simulink model "d_003_uc"  (Simulink 5.1)
settings: Solver=ode45  StartTime=0.0  StopTime=10.0  RelTol=1e-3
libraries: fm_lib x4
settings Model: Creator=fmilano  LastModifiedBy=fmilano  ExtModeAutoUpdateStatusClock=off  SignalLoggingName=logsout  BooleanDataType=on  RTWOptions="-aEnforceIntegerDowncast=1 -aFoldNonRolledExpr=1 -aInlineInvariantSignals=1 -aInlineParameters=0 -aLocalBlockOutputs=1 -aRollThreshold=5 -aZeroInternalMemoryAtStartup=1 -aZeroExternalMemoryAtStartup=1 -aInitFltsAndDblsToZero=1 -aForceBlockIOInitOptimize=0 -aGenerateReport=0 -aGenCodeOnly=0 -aRTWVerbose=1 -aIncludeHyperlinkInReport=0 -aLaunchReport=0 -aGenerateTraceInfo=0  -aForceParamTrailComments=0 -aGenerateComments=1 -aIgnoreCustomStorageClasses=1 -aIncHierarchyInIds=0 -aMaxRTWIdLen=31 -aShowEliminatedStatements=0 -aIncDataTypeInIds=0 -aInsertBlockDesc=0 -aIgnoreTestpoints=0 -aSimulinkBlockComments=1 -aInlinedPrmAccess=\"Literals\"  -aSuppressErrorStatus=0 -aModelReferenceCompliant=1 -aParenthesesLevel=\"Nominal\" -aModelStepFunctionPrototypeControlCompliant=0 -aPortableWordSizes=0 -aParMdlRefBuildCompliant=1 -aSupportNonInlinedSFcns=1 -aSupportContinuousTime=1 -aSupportComplex=1 -aSupportNonFinite=1 -aSupportAbsoluteTime=1 -aMultiwordLength=2048 -aTargetPreCompLibLocation=\"\" -aTargetLibSuffix=\"\" -aTargetFunctionLibrary=\"ANSI_C\" -aTargetFcnLib=\"ansi_tfl_tmw.mat\" -aMultiInstanceERTCode=0 -aLogVarNameModifier=\"rt_\" -aERTFirstTimeCompliant=0 -aIsPILTarget=0 -aCombineOutputUpdateFcns=0 -aGenerateASAP2=0 -aGenerateClassInterface=0 -aGenerateTestInterfaces=0 -aGenerateSampleERTMain=0 -aGenerateFullHeader=1 -aUtilityFuncGeneration=\"Auto\" -aIncludeFileDelimiter=\"Auto\" -aIncludeMdlTerminateFcn=1 -aPurelyIntegerCode=0 -aAutosarCompliant=0 -aERTCustomFileBanners=0 -aRTWCAPIStates=0 -aRTWCAPIParams=0 -aRTWCAPISignals=0 -aMatFileLogging=1 -aCompOptLevelCompliant=0 -aCPPClassGenCompliant=0 -aExtModeIntrfLevel=\"Level1\" -aExtModeMexFile=\"ext_comm\" -aExtModeTransport=0 -aExtModeStaticAllocSize=1000000 -aExtModeTesting=0 -aExtModeStaticAlloc=0 -aExtMode=0 -aERTMultiwordLength=256 -aERTMultiwordTypeDef=\"System defined\"  -aGenerateTraceInfo=0 -aIgnoreTestpoints=0 -aGenerateTraceInfo=0 -aGenerateTraceInfo=0 -aGenerateTraceInfo=0 -aGenerateTraceInfo=0 -aPrefixModelToSubsysFcnNames=1"

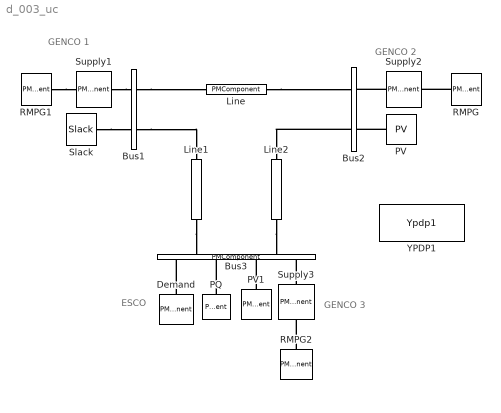
== system d_003_uc ==
  note: GENCO 1
  note: GENCO 2
  note: GENCO 3
  note: ESCO
  Bus1 : PMComponent  Tag=PSATblock  Description=Connection  PhysicalDomain=psatdomain  LeftPortType=p1  RightPortType=p1  LConnTagsString=__newl0|__newl1  RConnTagsString=__newr0|__newr1  mask(Bus){in=2, out=2, p2q=400, p3_4q=[1.00   0.00], p5q=1, p6q=1}
      mask prompts: in "Number of inputs:"; out "Number of outputs:"; p2q "Voltage Rating [kV]"; p3_4q "Voltage initial guess [p.u.  rad]"; p5q "Area number"; p6q "Region number"
      mask help: Bus block.
      mask init:
      | fm_inout
      mask CallbackString: ||||fm_block|
      mask Display: plot([0 1 1 0 0],[0 0 1 1 0])
  Bus2 : PMComponent  Tag=PSATblock  Description=Connection  PhysicalDomain=psatdomain  LeftPortType=p1  RightPortType=p1  LConnTagsString=__newl0|__newl1  RConnTagsString=__newr0|__newr1  mask(Bus){in=2, out=2, p2q=400, p3_4q=[1.00   0.00], p5q=2, p6q=1}
      mask prompts: in "Number of inputs:"; out "Number of outputs:"; p2q "Voltage Rating [kV]"; p3_4q "Voltage initial guess [p.u.  rad]"; p5q "Area number"; p6q "Region number"
      mask help: Bus block.
      mask init:
      | fm_inout
      mask CallbackString: ||||fm_block|
      mask Display: plot([0 1 1 0 0],[0 0 1 1 0])
  Bus3 : PMComponent  Tag=PSATblock  Description=Connection  Orientation=down  PhysicalDomain=psatdomain  LeftPortType=p1  RightPortType=p1  LConnTagsString=__newl0|__newl1  RConnTagsString=__newr0|__newr1|__newr2|__newr3  mask(Bus){in=2, out=4, p2q=400, p3_4q=[1.00  0.00], p5q=3, p6q=1}
      mask prompts: in "Number of inputs:"; out "Number of outputs:"; p2q "Voltage Rating [kV]"; p3_4q "Voltage initial guess [p.u.  rad]"; p5q "Area number"; p6q "Region number"
      mask help: Bus block.
      mask init:
      | fm_inout
      mask CallbackString: ||||fm_block|
      mask Display: plot([0 1 1 0 0],[0 0 1 1 0])
  Demand : PMComponent  Tag=PSATblock  Description=OPF & CPF  Orientation=down  PhysicalDomain=psatdomain  LeftPortType=p1  RightPortType=p1  LConnTagsString=__newl0  mask(Demand){p2q=100, p3q=1.00, p4q=0.60, p5_6q=[1.00  1.00], p8_9_10q=[0.00  0  0.00], p11_12_13q=[0.00  0.00  0.00], p14q=off, p15q=0, p16_17q=[0 0], out=0, p18q=on}
      mask prompts: p2q "Power Rating [MVA]"; p3q "Active Power [p.u.]"; p4q "Reactive Power [p.u.]"; p5_6q "Max and Min Power Demand [p.u.  p.u.]"; p8_9_10q "Cost = a + b*P + c*P^2 [$/h, $/MWh, $/(MW)^2 h]"; p11_12_13q "Cost = a + b*Q + c*Q^2 [$/h, $/MVArh, $/(MVAr)^2 h]"; p14q "Allow Unit Commitment"; p15q "Tie Breaking Cost [$/h]"; p16_17q "Up and down congestion costs [$/h $/h]"; out "Number of Output Signals"; p18q "Connected"
      mask help: This block defines a constant power load for bifurcation and market studies.
      mask init:
      | fm_inout;
      | [xs,ys]=fm_draw('$');
      mask StyleString: edit,edit,edit,edit,edit,edit,checkbox,edit,edit,popup(0|1),checkbox
      mask CallbackString: ||||||||||fm_block
      mask Display:
      | plot([ 1.0000    -0.5   -0.5  1],[ 0    0.866    -0.866    0])
      | color('blue')
      | plot(0.6*xs,0.6*ys)
  Line : PMComponent  Tag=PSATblock  Description=Power Flow  PhysicalDomain=psatdomain  LeftPortType=p1  RightPortType=p1  LConnTagsString=__newl0  RConnTagsString=__newr0  mask(Line){p3_4_5q=[100  400  60], p6q=0, p8q=0, p9q=0.10, p10q=0, p13_14_15q=[0.4  0.4  0.0], p16q=on}
      mask prompts: p3_4_5q "Power, Voltage and Frequency Ratings [MVA, kV, Hz]"; p6q "Length of line [km] (0 for p.u. parameters)"; p8q "Resistance [p.u. (Ohms/km)]"; p9q "Reactance [p.u. (H/km)]"; p10q "Susceptance [p.u. (F/km)]"; p13_14_15q "Imax, Pmax and Smax [p.u., p.u., p.u.]"; p16q "Connected"
      mask help: This block defines a pi model for a tree phase line.
      mask init:
      | [xp,yp] = fm_draw('pi');
      mask CallbackString: ||||||fm_block
      mask Display:
      | plot([-1  1  1 -1 -1],[-0.2 -0.2 0.2 0.2 -0.2])
      | color('blue')
      | plot(0.35*xp,0.2*yp)
  Line1 : PMComponent  Tag=PSATblock  Description=Power Flow  Orientation=down  PhysicalDomain=psatdomain  LeftPortType=p1  RightPortType=p1  LConnTagsString=__newl0  RConnTagsString=__newr0  mask(Line){p3_4_5q=[100  400  60], p6q=0, p8q=0, p9q=0.10, p10q=0, p13_14_15q=[0.4  0.4  0.0], p16q=on}
      mask prompts: p3_4_5q "Power, Voltage and Frequency Ratings [MVA, kV, Hz]"; p6q "Length of line [km] (0 for p.u. parameters)"; p8q "Resistance [p.u. (Ohms/km)]"; p9q "Reactance [p.u. (H/km)]"; p10q "Susceptance [p.u. (F/km)]"; p13_14_15q "Imax, Pmax and Smax [p.u., p.u., p.u.]"; p16q "Connected"
      mask help: This block defines a pi model for a tree phase line.
      mask init:
      | [xp,yp] = fm_draw('pi');
      mask CallbackString: ||||||fm_block
      mask Display:
      | plot([-1  1  1 -1 -1],[-0.2 -0.2 0.2 0.2 -0.2])
      | color('blue')
      | plot(0.35*xp,0.2*yp)
  Line2 : fm_lib/Power Flow/Line  Tag=PSATblock  Description=Power Flow  Orientation=down  PhysicalDomain=psatdomain  SubClassName=unknown  LeftPortType=p1  RightPortType=p1  LConnTagsString=__newl0  RConnTagsString=__newr0  p3_4_5q="[100  400  60]"  p6q=0  p8q=0  p9q=0.10  p10q=0  p13_14_15q="[0.4  0.4  0.0]"  p16q=on
  PQ : PMComponent  Tag=PSATblock  Description=Power Flow  Orientation=down  PhysicalDomain=psatdomain  LeftPortType=p1  RightPortType=p1  LConnTagsString=__newl0  mask(PQ){p2_3q=[100  400], p4_5q=[1.0 0.6], p6_7q=[1.2  0.8], p8q=on, p9q=on}
      mask prompts: p2_3q "Power and Voltage Ratings [MVA, kV]"; p4_5q "Active and Reactive Powers [p.u.  p.u.]"; p6_7q "Maximum and Minimum Allowable Voltage [p.u.   p.u.]"; p8q "Allow conversion to impendance for min & max voltage"; p9q "Connected"
      mask help:
      | This block defines a constant power load:
      |
      | P = Pcost.
      | Q = Qcost.
      mask CallbackString: |||fm_block|fm_block
      mask Display: plot([1 -0.5 -0.5 1],[0 0.866 -0.866 0])
  PV : fm_lib/Power Flow/PV  Tag=PSATblock  Description=Power Flow  Orientation=left  PhysicalDomain=psatdomain  SubClassName=unknown  LeftPortType=p1  RightPortType=p1  RConnTagsString=__newr0  p2_3q="[100  400]"  p4q=0.4  p5q=1.00  p6_7q="[0.8  -0.2]"  p8_9q="[1.1  0.9]"  p10q=1  p11q=on
  PV1 : PMComponent  Tag=PSATblock  Description=Power Flow  Orientation=up  PhysicalDomain=psatdomain  LeftPortType=p1  RightPortType=p1  RConnTagsString=__newr0  mask(PV){p2_3q=[100  400], p4q=0.4, p5q=1.00, p6_7q=[0.8  -0.2], p8_9q=[1.1  0.9], p10q=1, p11q=on}
      mask prompts: p2_3q "Power and Voltage Ratings [MVA, kV]"; p4q "Active Power [p.u.]"; p5q "Voltage Magnitude [p.u.]"; p6_7q "Qmax & Qmin [p.u.  p.u.]"; p8_9q "Vmax & Vmin [p.u.  p.u.]"; p10q "Loss Participation Factor"; p11q "Connected"
      mask help:
      | This block defines a PV bus for load flow studies:
      |
      | P = Pcost.
      | V = Vdes.
      mask init:
      | [x,y] = fm_draw('circle');
      | [xp,yp] = fm_draw('P');
      mask CallbackString: ||||||fm_block
      mask Display:
      | plot(x,y)
      | color('blue')
      | plot(0.3*xp-0.35,0.6*yp,[0.1 0.3 0.5],[0.3 -0.3 0.3])
  RMPG : PMComponent  Tag=PSATblock  Description=OPF & CPF  Orientation=left  PhysicalDomain=psatdomain  LeftPortType=p1  RightPortType=p1  RConnTagsString=__newr0  mask(Rmpg){p2q=100, p3_4q=[0.1  0.1], p5_6q=[2 2], p7_8q=[5 0], p9q=1, p10q=on}
      mask prompts: p2q "Power Rating [MVA]"; p3_4q "Ramp Up and Down Rates [p.u./h  p.u./h]"; p5_6q "Minimum Up and Down Times [h  h]"; p7_8q "Numbers of period up and down at initial time [h  h]"; p9q "Start Up Cost [$]"; p10q "Conneted"
      mask help: This block defines ramping parameters for generators for market studies.
      mask init:
      | [x,y] = fm_draw('circle');
      mask CallbackString: |||||fm_block
      mask Display:
      | plot(x,y)
      | color('blue')
      | plot([-0.5 0.5],[-0.4 -0.4],[-0.4 -0.4],[-0.45 0.4],[-0.4 0],[-0.5 0.3],[0 0.4],[0.3 0.3])
  RMPG1 : PMComponent  Tag=PSATblock  Description=OPF & CPF  PhysicalDomain=psatdomain  LeftPortType=p1  RightPortType=p1  RConnTagsString=__newr0  mask(Rmpg){p2q=100, p3_4q=[0.05 0.05], p5_6q=[2 2], p7_8q=[5 0], p9q=1, p10q=on}
      mask prompts: p2q "Power Rating [MVA]"; p3_4q "Ramp Up and Down Rates [p.u./h  p.u./h]"; p5_6q "Minimum Up and Down Times [h  h]"; p7_8q "Numbers of period up and down at initial time [h  h]"; p9q "Start Up Cost [$]"; p10q "Conneted"
      mask help: This block defines ramping parameters for generators for market studies.
      mask init:
      | [x,y] = fm_draw('circle');
      mask CallbackString: |||||fm_block
      mask Display:
      | plot(x,y)
      | color('blue')
      | plot([-0.5 0.5],[-0.4 -0.4],[-0.4 -0.4],[-0.45 0.4],[-0.4 0],[-0.5 0.3],[0 0.4],[0.3 0.3])
  RMPG2 : PMComponent  Tag=PSATblock  Description=OPF & CPF  Orientation=up  PhysicalDomain=psatdomain  LeftPortType=p1  RightPortType=p1  RConnTagsString=__newr0  mask(Rmpg){p2q=100, p3_4q=[0.15 0.15], p5_6q=[2 2], p7_8q=[0 5], p9q=1, p10q=on}
      mask prompts: p2q "Power Rating [MVA]"; p3_4q "Ramp Up and Down Rates [p.u./h  p.u./h]"; p5_6q "Minimum Up and Down Times [h  h]"; p7_8q "Numbers of period up and down at initial time [h  h]"; p9q "Start Up Cost [$]"; p10q "Conneted"
      mask help: This block defines ramping parameters for generators for market studies.
      mask init:
      | [x,y] = fm_draw('circle');
      mask CallbackString: |||||fm_block
      mask Display:
      | plot(x,y)
      | color('blue')
      | plot([-0.5 0.5],[-0.4 -0.4],[-0.4 -0.4],[-0.45 0.4],[-0.4 0],[-0.5 0.3],[0 0.4],[0.3 0.3])
  Slack : fm_lib/Power Flow/Slack  Tag=PSATblock  Description=Power Flow  PhysicalDomain=psatdomain  SubClassName=unknown  LeftPortType=p1  RightPortType=p1  RConnTagsString=__newr0  p2_3q="[100  400]"  p4q=1.00  p5q=0.00  p6_7q="[1.5  -1.5]"  p8_9q="[1.1  0.9]"  p10q=0.40  p11q=1  p12q=on  p13q=on
  Supply1 : PMComponent  Tag=PSATblock  Description=OPF & CPF  PhysicalDomain=psatdomain  LeftPortType=p1  RightPortType=p1  LConnTagsString=__newl0  RConnTagsString=__newr0  mask(Supply){p2q=100, p3q=0.0, p4_5q=[0.60 0.10], p7_8_9q=[6  9.8  0.1], p10_11_12q=[0.00  0.00  0.00], p13q=off, p14q=0, p15q=1, p16_17q=[1.5  -1.5], p18_19q=[0 0], in=1, p20q=on}
      mask prompts: p2q "Power Rating [MVA]"; p3q "Active Power [p.u.]"; p4_5q "Max and Min Power Supply [p.u.  p.u.]"; p7_8_9q "Cost = a + b*P + c*P^2 [$/h, $/MWh, $/(MW)^2 h]"; p10_11_12q "Cost = a + b*Q + c*Q^2 [$/h, $/MVArh, $/(MVAr)^2 h]"; p13q "Allow Unit Commitment"; p14q "Tie Breaking Cost [$/h]"; p15q "Loss participation factor"; p16_17q "Reactive power limits Qmax and Qmin [p.u. p.u.]"; p18_19q "Up and down congestion costs [$/h $/h]"; in "Number of Input Signals"; p20q "Connected"
      mask help: This block defines a PV bus for bifurcation and market studies:
      mask init:
      | fm_inout;
      | [x,y] = fm_draw('circle');
      | [xs,ys] = fm_draw('$');
      mask StyleString: edit,edit,edit,edit,edit,checkbox,edit,edit,edit,edit,popup(0|1|2),checkbox
      mask CallbackString: |||||||||||fm_block
      mask Display:
      | plot(x,y)
      | color('blue')
      | plot(xs,ys)
  Supply2 : PMComponent  Tag=PSATblock  Description=OPF & CPF  Orientation=left  PhysicalDomain=psatdomain  LeftPortType=p1  RightPortType=p1  LConnTagsString=__newl0  RConnTagsString=__newr0  mask(Supply){p2q=100, p3q=0.0, p4_5q=[0.60 0.10], p7_8_9q=[4  10.7  0.2], p10_11_12q=[0.00  0.00  0.00], p13q=off, p14q=0, p15q=1, p16_17q=[0.8  -0.2], p18_19q=[0 0], in=1, p20q=on}
      mask prompts: p2q "Power Rating [MVA]"; p3q "Active Power [p.u.]"; p4_5q "Max and Min Power Supply [p.u.  p.u.]"; p7_8_9q "Cost = a + b*P + c*P^2 [$/h, $/MWh, $/(MW)^2 h]"; p10_11_12q "Cost = a + b*Q + c*Q^2 [$/h, $/MVArh, $/(MVAr)^2 h]"; p13q "Allow Unit Commitment"; p14q "Tie Breaking Cost [$/h]"; p15q "Loss participation factor"; p16_17q "Reactive power limits Qmax and Qmin [p.u. p.u.]"; p18_19q "Up and down congestion costs [$/h $/h]"; in "Number of Input Signals"; p20q "Connected"
      mask help: This block defines a PV bus for bifurcation and market studies:
      mask init:
      | fm_inout;
      | [x,y] = fm_draw('circle');
      | [xs,ys] = fm_draw('$');
      mask StyleString: edit,edit,edit,edit,edit,checkbox,edit,edit,edit,edit,popup(0|1|2),checkbox
      mask CallbackString: |||||||||||fm_block
      mask Display:
      | plot(x,y)
      | color('blue')
      | plot(xs,ys)
  Supply3 : PMComponent  Tag=PSATblock  Description=OPF & CPF  Orientation=up  PhysicalDomain=psatdomain  LeftPortType=p1  RightPortType=p1  LConnTagsString=__newl0  RConnTagsString=__newr0  mask(Supply){p2q=100, p3q=0.0, p4_5q=[0.60 0.10], p7_8_9q=[8  12.6  0.25], p10_11_12q=[0.00  0.00  0.00], p13q=off, p14q=0, p15q=1, p16_17q=[0.8  -0.2], p18_19q=[0 0], in=1, p20q=on}
      mask prompts: p2q "Power Rating [MVA]"; p3q "Active Power [p.u.]"; p4_5q "Max and Min Power Supply [p.u.  p.u.]"; p7_8_9q "Cost = a + b*P + c*P^2 [$/h, $/MWh, $/(MW)^2 h]"; p10_11_12q "Cost = a + b*Q + c*Q^2 [$/h, $/MVArh, $/(MVAr)^2 h]"; p13q "Allow Unit Commitment"; p14q "Tie Breaking Cost [$/h]"; p15q "Loss participation factor"; p16_17q "Reactive power limits Qmax and Qmin [p.u. p.u.]"; p18_19q "Up and down congestion costs [$/h $/h]"; in "Number of Input Signals"; p20q "Connected"
      mask help: This block defines a PV bus for bifurcation and market studies:
      mask init:
      | fm_inout;
      | [x,y] = fm_draw('circle');
      | [xs,ys] = fm_draw('$');
      mask StyleString: edit,edit,edit,edit,edit,checkbox,edit,edit,edit,edit,popup(0|1|2),checkbox
      mask CallbackString: |||||||||||fm_block
      mask Display:
      | plot(x,y)
      | color('blue')
      | plot(xs,ys)
  YPDP1 : fm_lib/OPF & CPF/Ypdp1  Tag=PSATblock  Description=OPF & CPF  pxq=[55 75 100 120 100]
  connections:
  Line2/RConn1 -- Bus3/LConn2
  RMPG2/RConn1 -- Supply3/LConn1
  Line1/RConn1 -- Bus3/LConn1
  Bus1/RConn2 -- Line1/LConn1
  Bus1/RConn1 -- Line/LConn1
  Slack/RConn1 -- Bus1/LConn2
  RMPG1/RConn1 -- Supply1/LConn1
  Supply1/RConn1 -- Bus1/LConn1
  RMPG/RConn1 -- Supply2/LConn1
  Supply2/RConn1 -- Bus2/RConn1
  PV/RConn1 -- Bus2/RConn2
  Line/RConn1 -- Bus2/LConn1
  Bus2/LConn2 -- Line2/LConn1
  PV1/RConn1 -- Bus3/RConn3
  Supply3/RConn1 -- Bus3/RConn4
  Demand/LConn1 -- Bus3/RConn1
  PQ/LConn1 -- Bus3/RConn2
